simulink model "model_groundTethered"  (R2015b)
settings: Solver=ode45  StartTime=0.0  StopTime=T_sim  FixedStep=dt  RelTol=1e-3
PreLoadFcn:
  | setup;
InitFcn:
  | setup;
StartFcn:
  | setup;
values from neighbouring files (symbols this model uses):
  A_act = [-100 0 0 0 0 -100 0 0 0 0 -100 0 ... (16 elements, 4x4)]    [CD_spline.mat]    (also in CL_spline.mat; setup.m = -100*eye(4); setup_tmp_1p.m = -100*eye(4); setup_tmp_4p.m = -100*eye(4))
  A_init = [1.0386 0 12.9]    [CD_spline.mat]    (also in CL_spline.mat; setup_KiteModel_4points.m = Pc_init + d_n_r * w_k * w_rel * [-1;0;0])
  A_Kite = 7    [CD_spline.mat]    (also in CL_spline.mat; setup.m = 10.18; setup_tmp_1p.m = 10.18; setup_tmp_4p.m = 10.18)
  A_prd = [0 0 0 -640 0 0 0 0 0 0 -640 0 ... (36 elements, 6x6)]    [CD_spline.mat]    (also in CL_spline.mat; setup.m = 1000 * A_M_aug; setup_tmp_1p.m = 1000 * A_M_aug; setup_tmp_4p.m = 1000 * A_M_aug)
  A_ref = [0 0 0 -10000 0 0 0 0 0 0 -10000 0 ... (36 elements, 6x6)]    [CD_spline.mat]    (also in CL_spline.mat; setup.m = zeros(6); setup_tmp_1p.m = zeros(6); setup_tmp_4p.m = zeros(6))
  A_t_ref_cl = [0 0 0 -0.64 0 0 0 0 0 0 -0.64 0 ... (36 elements, 6x6)]    [CD_spline.mat]    (also in CL_spline.mat; setup.m = A_t_ref; setup_tmp_1p.m = A_t_ref; setup_tmp_4p.m = A_t_ref)
  alpha_0 = 10 * pi/180    (= 0.174532925199)    [setup_KiteModel_4points.m]
  alpha_s_0 = 10 * pi/180    (= 0.174532925199)    [setup_KiteModel_4points.m]
  ASideRel = 0    [CD_spline.mat]    (also in CL_spline.mat; setup.m; setup_tmp_1p.m; setup_tmp_4p.m = 0.306)
  B_act = [100 0 0 0 0 100 0 0 0 0 100 0 ... (16 elements, 4x4)]    [CD_spline.mat]    (also in CL_spline.mat; setup.m = 100*eye(4); setup_tmp_1p.m = 100*eye(4); setup_tmp_4p.m = 100*eye(4))
  B_init = [0 0 15.13]    [CD_spline.mat]    (also in CL_spline.mat; setup_KiteModel_4points.m = Pc_init + h_kite * [0;0;1;])
  B_ref = [0 0 0 10000 0 0 0 0 0 0 10000 0 ... (18 elements, 6x3)]    [CD_spline.mat]    (also in CL_spline.mat; setup.m = zeros(6,3); setup_tmp_1p.m = zeros(6,3); setup_tmp_4p.m = zeros(6,3))
  B_t_ref_cl = [0 0 0 0.64 0 0 0 0 0 0 0.64 0 ... (18 elements, 6x3)]    [CD_spline.mat]    (also in CL_spline.mat)
  Bpbl = [0 0 0 1 0 0 0 0 0 0 1 0 ... (18 elements, 6x3)]    [CD_spline.mat]    (also in CL_spline.mat; setup.m = [zeros(3); eye(3)]; setup_tmp_1p.m = [zeros(3); eye(3)]; setup_tmp_4p.m = [zeros(3); eye(3)])
  c0 = 614000    [CD_spline.mat]    (also in CL_spline.mat; setup.m; setup_tmp_1p.m; setup_tmp_4p.m)
  C_A = [0 0.3 -1e-06 1 -0.3 0 1e-06 1 0 -0.3 -1e-06 1 ... (16 elements, 4x4)]    [CD_spline.mat]    (also in CL_spline.mat; setup.m = [0, -R, 0, R; setup_tmp_1p.m = [0, -R, 0, R; setup_tmp_4p.m = [0, -R, 0, R)
  C_A_inv = [0 -1.66666666667 -1.23358113847e-17 1.66666666667 1.66666666667 2.46716227694e-17 -1.66666666667 0 -250000 250000 -250000 250000 ... (16 elements, 4x4)]    [CD_spline.mat]    (also in CL_spline.mat; setup.m = C_A \eye(4); setup_tmp_1p.m = C_A \eye(4); setup_tmp_4p.m = C_A \eye(4))
  C_D_Kite = 0.05    [CD_spline.mat]    (also in CL_spline.mat; setup.m = 0.005; setup_tmp_1p.m = 0.005)
  C_init = [0 2.5965 12.9]    [CD_spline.mat]    (also in CL_spline.mat; setup_KiteModel_4points.m = Pc_init + 0.5 * w_k * w_rel * [0;1;0])
  C_L_Kite = 0.1    [CD_spline.mat]    (also in CL_spline.mat; setup.m = 0.01; setup_tmp_1p.m = 0.01)
  CD_spline_coefs = CD_spline.coefs    [setup_KiteModel_4points.m]
  CD_tether = 0.96    [CD_spline.mat]    (also in CL_spline.mat; setup.m; setup_tmp_1p.m; setup_tmp_4p.m)
  CL_spline_coefs = CL_spline.coefs    [setup_KiteModel_4points.m]
  d0 = 473    [CD_spline.mat]    (also in CL_spline.mat; setup.m; setup_tmp_1p.m; setup_tmp_4p.m)
  D_init = [0 -2.5965 12.9]    [CD_spline.mat]    (also in CL_spline.mat; setup_KiteModel_4points.m = Pc_init - 0.5 * w_k * w_rel * [0;1;0])
  d_tether = 0.004    [CD_spline.mat]    (also in CL_spline.mat; setup.m; setup_tmp_1p.m; setup_tmp_4p.m)
  delta_dead = 0.5    [CD_spline.mat]    (also in CL_spline.mat; setup.m; setup_tmp_1p.m; setup_tmp_4p.m)
  e_0 = 0.01    [CD_spline.mat]    (also in CL_spline.mat; setup.m; setup_tmp_1p.m; setup_tmp_4p.m)
  epsilon = 0.6    [CD_spline.mat]    (also in CL_spline.mat; setup.m; setup_tmp_1p.m; setup_tmp_4p.m)
  eta_init = [0 0 0]    [CD_spline.mat]    (also in CL_spline.mat; setup.m = zeros(3,1); setup_tmp_1p.m = zeros(3,1); setup_tmp_4p.m = zeros(3,1))
  g = 9.81    [CD_spline.mat]    (also in CL_spline.mat; setup.m; setup_tmp_1p.m; setup_tmp_4p.m)
  g_vec = [0 0 9.81]    [CD_spline.mat]    (also in CL_spline.mat; setup.m = [0;0;9.81]; setup_tmp_1p.m = [0;0;9.81]; setup_tmp_4p.m = [0;0;9.81])
  Gamma_ad = 100    [CD_spline.mat]    (also in CL_spline.mat; setup.m = 100;100; setup_tmp_1p.m = 100;100; setup_tmp_4p.m = 100;100)
  Gamma_pred = 100    [CD_spline.mat]    (also in CL_spline.mat; setup.m; setup_tmp_1p.m; setup_tmp_4p.m)
  J = [0.018  0  0; 0  0.018  0; 0  0  0.009]    [CD_spline.mat]    (also in CL_spline.mat; setup.m = diag([Ixx, Iyy, Izz]); setup_tmp_1p.m = diag([Ixx, Iyy, Izz]); setup_tmp_4p.m = diag([Ixx, Iyy, Izz]))
  Jinv = [55.5555555556  0  0; 0  55.5555555556  0; 0  0  111.111111111]    [CD_spline.mat]    (also in CL_spline.mat; setup.m = J \ eye(3); setup_tmp_1p.m = J \ eye(3); setup_tmp_4p.m = J \ eye(3))
  K = 1 - ASideRel    [setup_KiteModel_4points.m]
  k_e_eta = 10000    [CD_spline.mat]    (also in CL_spline.mat; setup.m; setup_tmp_1p.m; setup_tmp_4p.m)
  k_e_eta_dot = 400    [CD_spline.mat]    (also in CL_spline.mat; setup.m; setup_tmp_1p.m; setup_tmp_4p.m)
  k_e_eta_I = 1    [CD_spline.mat]    (also in CL_spline.mat; setup.m; setup_tmp_1p.m; setup_tmp_4p.m)
  K_i_t = [10  0  0; 0  10  0; 0  0  10]    [CD_spline.mat]    (also in CL_spline.mat; setup.m = 10*eye(3); setup_tmp_1p.m = 10*eye(3); setup_tmp_4p.m = 10*eye(3))
  K_v_t = [1.6  0  0; 0  1.6  0; 0  0  1.6]    [CD_spline.mat]    (also in CL_spline.mat; setup.m = 2*omega_0_trans*zeta_0_trans*eye(3); setup_tmp_1p.m = 2*omega_0_trans*zeta_0_trans*eye(3); setup_tmp_4p.m = 2*omega_0_trans*zeta_0_trans*eye(3))
  K_x_t = [0.64  0  0; 0  0.64  0; 0  0  0.64]    [CD_spline.mat]    (also in CL_spline.mat; setup.m = omega_0_trans^2*eye(3); setup_tmp_1p.m = omega_0_trans^2*eye(3); setup_tmp_4p.m = omega_0_trans^2*eye(3))
  l_s0 = 1    [CD_spline.mat]    (also in CL_spline.mat; setup.m = 1.42857142857; setup_tmp_1p.m = 1.42857142857; setup_tmp_4p.m = 1.66666666667)
  l_s_BP = norm( B_init - p_B_UAV_init)    [setup_KiteModel_4points.m]
  l_s_PUav = norm( pos_UAV_init - p_B_UAV_init)    [setup_KiteModel_4points.m]
  ls_AB = norm( A_init -  B_init)    [setup_KiteModel_4points.m]
  ls_AC = norm( A_init -  C_init)    [setup_KiteModel_4points.m]
  ls_AD = norm( A_init -  D_init)    [setup_KiteModel_4points.m]
  ls_AKcu = norm( A_init -  P_kcu)    [setup_KiteModel_4points.m]
  ls_CB = norm( C_init -  B_init)    [setup_KiteModel_4points.m]
  ls_CD = norm( C_init -  D_init)    [setup_KiteModel_4points.m]
  ls_CKcu = norm( C_init - P_kcu)    [setup_KiteModel_4points.m]
  ls_DB = norm( D_init - B_init )    [setup_KiteModel_4points.m]
  ls_DKcu = norm( D_init - P_kcu)    [setup_KiteModel_4points.m]
  m_A = 3.29    [CD_spline.mat]    (also in CL_spline.mat; setup_KiteModel_4points.m = nose_mass_fraction * m_kite)
  m_B = 1.484    [CD_spline.mat]    (also in CL_spline.mat; setup_KiteModel_4points.m = 0.4 * (1-nose_mass_fraction)*m_kite)
  m_C = 1.113    [CD_spline.mat]    (also in CL_spline.mat; setup_KiteModel_4points.m = 0.3 * (1-nose_mass_fraction)*m_kite)
  m_D = 1.113    [CD_spline.mat]    (also in CL_spline.mat; setup_KiteModel_4points.m = 0.3 * (1-nose_mass_fraction)*m_kite)
  m_kite = 7    [CD_spline.mat]    (also in CL_spline.mat; setup.m = 5;7; setup_tmp_1p.m = 5;7; setup_tmp_4p.m = 6.21)
  m_p = 0.013    [CD_spline.mat]    (also in CL_spline.mat; setup.m = 0.0185714285714; setup_tmp_1p.m = 0.0185714285714; setup_tmp_4p.m = 0.0216666666667)
  m_uav = 3    [CD_spline.mat]    (also in CL_spline.mat; setup.m; setup_tmp_1p.m; setup_tmp_4p.m)
  n = 10    [CD_spline.mat]    (also in CL_spline.mat; setup.m; setup_tmp_1p.m; setup_tmp_4p.m)
  n_t_p = 7    [setup.m]    (also in setup_tmp_1p.m; setup_tmp_4p.m = 6)
  omega_init = [0 0 0]    [CD_spline.mat]    (also in CL_spline.mat; setup.m = zeros(3,1); setup_tmp_1p.m = zeros(3,1); setup_tmp_4p.m = zeros(3,1))
  p_B_UAV_init = B_init + [0;0;l_s0]    [setup_KiteModel_4points.m]
  p_init = [0 0 1 0 0 2 0 0 3 0 0 4 ... (30 elements, 30x1)]    [CD_spline.mat]    (also in CL_spline.mat; setup.m = zeros(3*n,1); setup_tmp_1p.m = zeros(3*n,1); setup_tmp_4p.m = zeros(3*n,1))
  p_init_4p = zeros(3*n_t_p,1)    [setup.m]    (also in setup_tmp_4p.m)
  P_prd = [712.5 0 0 156.25 0 0 0 712.5 0 0 156.25 0 ... (36 elements, 6x6)]    [CD_spline.mat]    (also in CL_spline.mat; setup.m = 1000 * P_tref; setup_tmp_1p.m = 1000 * P_tref; setup_tmp_4p.m = 1000 * P_tref)
  P_tref = [0.7125 0 0 0.15625 0 0 0 0.7125 0 0 0.15625 0 ... (36 elements, 6x6)]    [CD_spline.mat]    (also in CL_spline.mat; setup.m = lyap(A_M_aug', Q); setup_tmp_1p.m = lyap(A_M_aug', Q); setup_tmp_4p.m = lyap(A_M_aug', Q))
  pos_UAV_init = p_B_UAV_init + [0;0;l_s0]    [setup_KiteModel_4points.m]
  rho_air = 1.225    [CD_spline.mat]    (also in CL_spline.mat; setup.m; setup_tmp_1p.m; setup_tmp_4p.m)
  rho_t = 0.013    [CD_spline.mat]    (also in CL_spline.mat; setup.m; setup_tmp_1p.m; setup_tmp_4p.m)
  sample_log = 0.01    [CD_spline.mat]    (also in CL_spline.mat; setup.m; setup_tmp_1p.m; setup_tmp_4p.m)
  t0 = 1    [CD_spline.mat]    (also in CL_spline.mat; setup.m; setup_tmp_1p.m; setup_tmp_4p.m)
  t1 = 3    [CD_spline.mat]    (also in CL_spline.mat; setup.m; setup_tmp_1p.m; setup_tmp_4p.m)
  T_launch = 40    [CD_spline.mat]    (also in CL_spline.mat; setup.m; setup_tmp_1p.m; setup_tmp_4p.m)
  Theta_max = 60    [CD_spline.mat]    (also in CL_spline.mat; setup.m; setup_tmp_1p.m; setup_tmp_4p.m)
  Thrust_Max = 80    [CD_spline.mat]    (also in CL_spline.mat; setup.m = 1000000000; setup_tmp_1p.m = 100; setup_tmp_4p.m = 1000000000)
  Tx = 10    [CD_spline.mat]    (also in CL_spline.mat; setup.m; setup_tmp_1p.m; setup_tmp_4p.m)
  Ty = 10    [CD_spline.mat]    (also in CL_spline.mat; setup.m; setup_tmp_1p.m; setup_tmp_4p.m)
  Tz = 10    [CD_spline.mat]    (also in CL_spline.mat; setup.m; setup_tmp_1p.m; setup_tmp_4p.m = 15)
  v_w_vec = [1 1 1]    [CD_spline.mat]    (also in CL_spline.mat; setup.m = [0.1;0;0]; setup_tmp_1p.m = [1;0;0]; setup_tmp_4p.m = [3;0;0])
  x0num = 0    [CD_spline.mat]    (also in CL_spline.mat; polynomial_trajectory.m = double( solutions_x.x0 ))
  x1num = 0    [CD_spline.mat]    (also in CL_spline.mat; polynomial_trajectory.m = double( solutions_x.x1 ))
  x2num = 0    [CD_spline.mat]    (also in CL_spline.mat; polynomial_trajectory.m = double( solutions_x.x2 ))
  x3num = 0.05    [CD_spline.mat]    (also in CL_spline.mat; polynomial_trajectory.m = double( solutions_x.x3 ))
  x4num = -0.0075    [CD_spline.mat]    (also in CL_spline.mat; polynomial_trajectory.m = double( solutions_x.x4 ))
  x5num = 0.0003    [CD_spline.mat]    (also in CL_spline.mat; polynomial_trajectory.m = double( solutions_x.x5 ))
  x_drone_init = [0 0 10]    [CD_spline.mat]    (also in CL_spline.mat; setup.m = p_init(3*n-2:3*n); setup_KiteModel_4points.m = pos_UAV_init; setup_tmp_1p.m = p_init(3*n-2:3*n))
  xT = 5    [CD_spline.mat]    (also in CL_spline.mat; setup.m = 1; setup_tmp_1p.m = 10; setup_tmp_4p.m = 10)
  y0num = 0    [CD_spline.mat]    (also in CL_spline.mat; polynomial_trajectory.m = double( solutions_y.y0 ))
  y1num = 0    [CD_spline.mat]    (also in CL_spline.mat; polynomial_trajectory.m = double( solutions_y.y1 ))
  y2num = 0    [CD_spline.mat]    (also in CL_spline.mat; polynomial_trajectory.m = double( solutions_y.y2 ))
  y3num = 0.1    [CD_spline.mat]    (also in CL_spline.mat; polynomial_trajectory.m = double( solutions_y.y3 ))
  y4num = -0.015    [CD_spline.mat]    (also in CL_spline.mat; polynomial_trajectory.m = double( solutions_y.y4 ))
  y5num = 0.0006    [CD_spline.mat]    (also in CL_spline.mat; polynomial_trajectory.m = double( solutions_y.y5 ))
  yT = 10    [CD_spline.mat]    (also in CL_spline.mat; setup.m = 1; setup_tmp_1p.m = 0; setup_tmp_4p.m = 0)
  z0num = 10    [CD_spline.mat]    (also in CL_spline.mat; polynomial_trajectory.m = double( solutions_z.z0 ))
  z1num = 0    [CD_spline.mat]    (also in CL_spline.mat; polynomial_trajectory.m = double( solutions_z.z1 ))
  z2num = 0    [CD_spline.mat]    (also in CL_spline.mat; polynomial_trajectory.m = double( solutions_z.z2 ))
  z3num = 0.4    [CD_spline.mat]    (also in CL_spline.mat; polynomial_trajectory.m = double( solutions_z.z3 ))
  z4num = -0.06    [CD_spline.mat]    (also in CL_spline.mat; polynomial_trajectory.m = double( solutions_z.z4 ))
  z5num = 0.0024    [CD_spline.mat]    (also in CL_spline.mat; polynomial_trajectory.m = double( solutions_z.z5 ))
  zT = 50    [CD_spline.mat]    (also in CL_spline.mat; setup.m; setup_tmp_1p.m; setup_tmp_4p.m = 75)
libraries: simulink x1
(part 3 of 3)

== matlab function model_groundTethered/Controller/Outer_Loop_Position/Adaptive_Augmentation/Proj(Theta_hat, GammaY)_multicolumns/Projection_Input_1/calculate_gradf ==
  data: theta_hat input; gradf output; Theta_max input; epsilon input
function gradf = fcn(theta_hat,Theta_max, epsilon )
%#codegen
gradf = ( 2*(1+epsilon) ) / (epsilon*(Theta_max)^2) * theta_hat ;

== matlab function model_groundTethered/Controller/Pseudo_Control_Hedging/Rotate thrust vector according to attitude ==
  data: u_Thrust_I input; eta input; u_Thrust_B output
function u_Thrust_B   = thrust_Bz_direction(  u_Thrust_I, eta) 

phi = eta(1); 
theta = eta(2); 
psi = eta(3); 

% Rotate thrust vector such that it is perpendicular to the "rotor blades"
u_Thrust_B = [cos(psi)*cos(theta), sin(psi)*cos(theta), -sin(theta); 
            cos(psi)*sin(theta)*sin(phi)-sin(psi)*cos(phi), sin(psi)*sin(theta)*sin(phi)+cos(psi)*cos(phi), cos(theta)*sin(phi); 
            cos(psi)*sin(theta)*cos(phi)+sin(psi)*sin(phi), sin(psi)*sin(theta)*cos(phi)-cos(psi)*sin(phi), cos(theta)*cos(phi)] *...
            [0;0;u_Thrust_I];

== matlab function model_groundTethered/Controller/Pseudo_Control_Hedging/Plant_Inversion_RD2_backwards/Plant_Inversion ==
  data: omega input; nu_tot_rot_hat output; eta input; eta_dot input; J parameter; Jinv parameter; M_hat input
function nu_tot_rot_hat = fcn(omega, eta, eta_dot,J, Jinv, M_hat)
%#codegen
p = omega(1); 
q = omega(2); 
r = omega(3); 
Ix = J(1,1); 
Iy = J(2,2); 
Iz = J(3,3); 


cross_coupling = [ Iy*q*r - Iz*q*r
 Iz*p*r - Ix*p*r;
 Ix*p*q - Iy*p*q];

% T_inv = [1, sin(eta(1)) * tan(eta(2)), cos(eta(1)) * tan(eta(2)) ; 
% 0, cos(eta(1)), -sin(eta(1)); 
% 0, sin(eta(1))/cos(eta(2)), cos(eta(1))/cos(eta(2))] \ eye(3); 

T = [1, sin(eta(1)) * tan(eta(2)), cos(eta(1)) * tan(eta(2)) ; 
0, cos(eta(1)), -sin(eta(1)); 
0, sin(eta(1))/cos(eta(2)), cos(eta(1))/cos(eta(2))];

T_dot = eta_dot(1) * [0, cos(eta(1)) * tan(eta(2)), -sin(eta(1))*tan(eta(2)); 
                      0, -sin(eta(1)), -cos(eta(1));
                      0, cos(eta(1))/cos(eta(2)), -sin(eta(1))/cos(eta(2))]+...
        eta_dot(2) * [0, sin(eta(1))/cos(eta(2))^2, cos(eta(1))/cos(eta(2))^2; 
                       0, 0, 0; 
                       0, sin(eta(1))*sin(eta(2))/cos(eta(2))^2, cos(eta(1))*sin(eta(2))/cos(eta(2))^2];
                          
%u_NDI = -cross_coupling + J * T_inv * ( -T_dot * omega + nu_tot); 

nu_tot_rot_hat = T * Jinv * ( M_hat + cross_coupling ) + T_dot *omega;

== matlab function model_groundTethered/Controller/Pseudo_Control_Hedging/Plant_Inversion_RD2_backwards/estimate_eta_dot ==
  data: omega input; eta input; eta_dot output
function eta_dot  = fcn( omega, eta)
%#codegen

eta_dot = [1, sin(eta(1)) * tan(eta(2)), cos(eta(1)) * tan(eta(2)) ; 
0, cos(eta(1)), -sin(eta(1)); 
0, sin(eta(1))/cos(eta(2)), cos(eta(1))/cos(eta(2))] * omega;

== matlab function model_groundTethered/Controller/Outer_Loop_Position/Adaptive_Augmentation/Smooth_Deadzone_MRAC/smooth_deadzone ==
  data: e_norm input; mu_dead output; delta_dead input; e_0 input
function mu_dead = fcn(e_norm, delta_dead, e_0)
%#codegen

mu_dead = max( 0, min( 1, (e_norm - delta_dead*e_0)/...
                          ( (1-delta_dead) * e_0) ) );

== matlab function model_groundTethered/Controller/Outer_Loop_Position/Calc_Ref_Attitude ==
  data: T_ref input; Eta_Cmd output; eta input
function Eta_Cmd  = fcn(T_ref, eta)
%#codegen
psi = eta(3); 
theta = eta(2); 
phi = eta(1); 

psi_c = 0;

T = norm( T_ref ); 

phi_c = -asin( 1/T * (T_ref(1) * sin(psi_c) - T_ref(2) * cos(psi_c)) ); 
theta_c = -atan( 1/T_ref(3) * (T_ref(1) * cos(psi_c) + T_ref(2) * sin(psi_c))); 

Eta_Cmd = [phi_c;theta_c; 0];

== matlab function model_groundTethered/Plant/Tether_Kite_Tether_UAV_Dynamics_4P/Kite_Model_4p/Kite_Model_4p ==
  data: x_dotdot_kite output; v_w_vec input; ASideRel parameter; alpha_d input; alpha_0 parameter; alpha_s input; alpha_s_0 parameter; x_kite_A input; x_kite_B input; x_kite_C input; x_kite_D input; x_kite_kcu input; x_above_kite input; xdot_kite_A input; xdot_kite_B input; xdot_kite_C input; xdot_kite_D input; xdot_kite_kcu input; xdot_above_kite input; CL_spline_coefs parameter; CD_spline_coefs parameter; rho_air parameter; A_Kite parameter; K parameter; g_vec parameter; m_A parameter; m_B parameter; m_C parameter; m_D parameter; d0 parameter; c0 parameter; ls_AC parameter; ls_AB parameter; ls_AKcu parameter; ls_AD parameter; ls_CB parameter; ls_CD parameter; ls_CKcu parameter; ls_DKcu parameter; ls_DB parameter; l_s_BP parameter
%% 4 Point kite implementation

function x_dotdot_kite  = fcn( v_w_vec, ASideRel, alpha_d,alpha_0,alpha_s, alpha_s_0,...
    x_kite_A, x_kite_B, x_kite_C, x_kite_D, x_kite_kcu,...
    x_above_kite, xdot_kite_A, xdot_kite_B, xdot_kite_C, xdot_kite_D,xdot_kite_kcu,xdot_above_kite,...
    CL_spline_coefs, CD_spline_coefs, rho_air, A_Kite,K,g_vec, m_A, m_B, m_C, m_D, d0, c0,...
    ls_AC, ls_AB, ls_AKcu, ls_AD, ls_CB, ls_CD, ls_CKcu, ls_DKcu, ls_DB,l_s_BP )


% Calculation of unity vectors of the kite body fixed frame
x_kite_Pc = 0.5 * (x_kite_C + x_kite_D);
e_z_k = (x_kite_Pc - x_kite_B)/sqrt((x_kite_Pc - x_kite_B)'*(x_kite_Pc - x_kite_B));
e_y_k = (x_kite_C - x_kite_D)/sqrt((x_kite_C - x_kite_D)'*(x_kite_C - x_kite_D));
e_x_k = [ e_y_k(2)*e_z_k(3) - e_y_k(3)*e_z_k(2);
    e_y_k(3)*e_z_k(1) - e_y_k(1)*e_z_k(3);
    e_y_k(1)*e_z_k(2) - e_y_k(2)*e_z_k(1)];

% Calculation of the apparent wind speeds at the 3 lifting surfaces
v_a_k_B = v_w_vec - xdot_kite_B;
v_a_k_C = v_w_vec - xdot_kite_C;
v_a_k_D = v_w_vec - xdot_kite_D;

% Calculation of the apparent wind speeds in xy and xz plane
v_a_B_xz = v_a_k_B - (v_a_k_B'*e_y_k)*e_y_k;
v_a_C_xy = v_a_k_C - (v_a_k_C'*e_z_k)*e_z_k;
v_a_D_xy = v_a_k_D - (v_a_k_D'*e_z_k)*e_z_k;

% Calculation of angles of attack
alpha_B  = pi - acos( (v_a_B_xz'*e_x_k)/sqrt(v_a_B_xz'*v_a_B_xz) ) - alpha_d + alpha_0;
alpha_C  = pi - acos( (v_a_C_xy'*e_x_k)/sqrt(v_a_C_xy'*v_a_C_xy) ) - alpha_s + alpha_s_0;
alpha_D  = pi - acos( (v_a_D_xy'*e_x_k)/sqrt(v_a_D_xy'*v_a_D_xy) ) + alpha_s + alpha_s_0;

% Calculation of Cl(alpha)_i and Cd(alpha)_i based on the spline
% coefficients
[ C_L_B, C_D_B ] = calcCLandCD_4pKite( alpha_B,CL_spline_coefs,CD_spline_coefs );
[ C_L_C, C_D_C ] = calcCLandCD_4pKite( alpha_C,CL_spline_coefs,CD_spline_coefs );
[ C_L_D, C_D_D ] = calcCLandCD_4pKite( alpha_D,CL_spline_coefs,CD_spline_coefs);

% Calculate the lift and drag forces of the lifting surfaces
[ F_L_B, F_L_C, F_L_D,...
    F_D_B, F_D_C, F_D_D  ] = calc4pKiteForces( C_L_B,C_L_C,C_L_D,...
    C_D_B, C_D_C, C_D_D,...
    rho_air, A_Kite, ASideRel,K,...
    e_y_k, e_z_k,...
    v_a_k_B, v_a_k_C, v_a_k_D, ...
    v_a_B_xz, v_a_C_xy, v_a_D_xy);

% Spring-Damper forces 
% Constant bridle line (as defined in the setup_KiteModel_4points.m script)
% Notation: z.B. AC => x_A - x_C => belongs to forces of inertia

c = c0;
d = d0;

f_AC = calcSpringDamperForce(c, norm(x_kite_A-x_kite_C) , ls_AC, d, x_kite_A - x_kite_C, xdot_kite_A - xdot_kite_C, 1 );
f_AB = calcSpringDamperForce(c, norm(x_kite_A-x_kite_B) , ls_AB, d, x_kite_A - x_kite_B, xdot_kite_A - xdot_kite_B, 1 );
f_AD = calcSpringDamperForce(c, norm(x_kite_A-x_kite_D) , ls_AD, d, x_kite_A - x_kite_D, xdot_kite_A - xdot_kite_D, 1 );
f_A_kcu = calcSpringDamperForce(c, norm(x_kite_A-x_kite_kcu) , ls_AKcu, d, x_kite_A - x_kite_kcu, xdot_kite_A - xdot_kite_kcu, 1 );
f_CA = -f_AC; 
f_CD = calcSpringDamperForce(c, norm(x_kite_C-x_kite_D) , ls_CD, d, x_kite_C - x_kite_D, xdot_kite_C - xdot_kite_D, 1 ); 
f_CB = calcSpringDamperForce(c, norm(x_kite_C-x_kite_B) , ls_CB, d, x_kite_C - x_kite_B, xdot_kite_C - xdot_kite_B, 1 ); 
f_C_kcu = calcSpringDamperForce(c, norm(x_kite_C-x_kite_kcu) , ls_CKcu, d, x_kite_C - x_kite_kcu, xdot_kite_C - xdot_kite_kcu, 1 );
f_DA = -f_AD; 
f_DC = -f_CD; 
f_DB = calcSpringDamperForce(c, norm(x_kite_D-x_kite_B) , ls_DB, d, x_kite_D - x_kite_B, xdot_kite_D - xdot_kite_B, 1 ); 
f_D_kcu = calcSpringDamperForce(c, norm(x_kite_D-x_kite_kcu) , ls_DKcu, d, x_kite_D - x_kite_kcu, xdot_kite_D - xdot_kite_kcu, 1 );
f_BA = -f_AB; 
f_BC = -f_CB; 
f_BD = -f_DB;  
f_above_kite = calcSpringDamperForce(c0, norm(x_above_kite-x_kite_B) , l_s_BP, d0, x_above_kite - x_kite_B, xdot_above_kite - xdot_kite_B, 1 ); 

x_kite_A_dotdot = 1/m_A*( - m_A*g_vec - f_AC - f_AB - f_A_kcu );
x_kite_B_dotdot = 1/m_B*(F_L_B + F_D_B - m_B*g_vec - f_BA - f_BC - f_BD + f_above_kite  );
x_kite_C_dotdot = 1/m_C*(F_L_C + F_D_C - m_C*g_vec - f_CA - f_CD - f_CB - f_C_kcu );
x_kite_D_dotdot = 1/m_D*(F_L_D + F_D_D - m_D*g_vec - f_DA - f_DC - f_DB - f_D_kcu );

x_dotdot_kite = [x_kite_A_dotdot;
                 x_kite_B_dotdot;
                 x_kite_C_dotdot;
                 x_kite_D_dotdot];

end

== matlab function model_groundTethered/Plant/Tether_Kite_Tether_UAV_Dynamics_1P/Kite_Model_1P/Kite_Model ==
  data: launch_flag input; x_dotdot_kite output; rho_air parameter; A_Kite parameter; g_vec parameter; C_L_Kite parameter; C_D_Kite parameter; m_kite parameter; v_w_vec input; ASideRel parameter; xp_aboveKite input; x_kite input; xp_belowKite input; xdot_aboveKite input; xdot_kite input; xdot_belowKite input; l_s input; c0 parameter; d0 parameter; l_s0 parameter
function x_dotdot_kite  = fcn(launch_flag,...
    rho_air, A_Kite, g_vec, C_L_Kite, C_D_Kite, m_kite, v_w_vec, ASideRel,...
    xp_aboveKite, x_kite, xp_belowKite,xdot_aboveKite, xdot_kite,...
    xdot_belowKite, l_s, c0, d0, l_s0)

c = c0/l_s;
d = d0/l_s;

% Tether forces from below and above
f_T_below = calcSpringDamperForce(c, norm(x_kite-xp_belowKite) , l_s, d, x_kite - xp_belowKite, xdot_kite - xdot_belowKite, 1 );
f_T_above = calcSpringDamperForce(c0, norm(xp_aboveKite-x_kite), l_s0, d0, xp_aboveKite-x_kite, xdot_aboveKite - xdot_kite, 1 );

% Calculate the apparent wind speed
v_a_k = v_w_vec - xdot_kite;
if launch_flag
    C_L_Kite = 0.5;
    C_D_Kite = 0.2;
end

[L_kite, D_kite, S_kite] = calcKiteForces(x_kite, xp_belowKite, ...
                                        v_a_k, C_L_Kite, rho_air, A_Kite, C_D_Kite, ASideRel);
m_kite = 0.1;
if launch_flag % kite is launched
    x_dotdot_kite = 1/m_kite * ( -f_T_below  - m_kite*g_vec  ... % remove the conection to 'drone tether'
        + D_kite + L_kite + 0*S_kite ) ;  % Kite dynamics
else
    x_dotdot_kite = 1/m_kite * ( -f_T_below + f_T_above - m_kite*g_vec  ...
        + 0*D_kite + 0*L_kite  + 0*S_kite);  % Kite dynamics
end

== matlab function model_groundTethered/Plant/Tether_Kite_Tether_UAV_Dynamics_4P/UAV_Model/Rotate thrust vector according to attitude ==
  data: u_Thrust_I input; eta input; u_Thrust_B output
function u_Thrust_B   = thrust_Bz_direction(  u_Thrust_I, eta) 

phi = eta(1); 
theta = eta(2); 
psi = eta(3); 

% Rotate thrust vector such that it is perpendicular to the "rotor blades"
u_Thrust_B = [cos(psi)*cos(theta), sin(psi)*cos(theta), -sin(theta); 
            cos(psi)*sin(theta)*sin(phi)-sin(psi)*cos(phi), sin(psi)*sin(theta)*sin(phi)+cos(psi)*cos(phi), cos(theta)*sin(phi); 
            cos(psi)*sin(theta)*cos(phi)+sin(psi)*sin(phi), sin(psi)*sin(theta)*cos(phi)-cos(psi)*sin(phi), cos(theta)*cos(phi)] *...
            [0;0;u_Thrust_I];

== matlab function model_groundTethered/Controller/Outer_Loop_Position/Adaptive_Augmentation/Proj(Theta_hat, GammaY)_1column/Proj(Theta,Theta_dot) ==
  data: flag output; f input; gradf input; Theta_dot input; Theta_hat_dot_ output; direction output; orthogonal_part output
function  [flag,Theta_hat_dot_, direction, orthogonal_part] = fcn(f, gradf, Theta_dot )
%#codegen


if ( f > 0 && Theta_dot'*gradf > 0 )
    flag  = 1;
    direction = Theta_dot'*gradf;
    Theta_hat_dot_ = Theta_dot - f * ( (gradf*gradf') / (gradf'*gradf) * Theta_dot )   ;
    orthogonal_part = f * ( (gradf*gradf') / (gradf'*gradf) * Theta_dot );
else
    direction = Theta_dot'*gradf;
    flag = 0;
    Theta_hat_dot_ =  Theta_dot;
    orthogonal_part = zeros(3,1);
end

== matlab function model_groundTethered/Controller/Outer_Loop_Position/Adaptive_Augmentation/Proj(Theta_hat, GammaY)_1column/calculate_f ==
  data: theta_hat input; f output; Theta_max input; epsilon input
function f   = fcn(theta_hat,Theta_max, epsilon )
%#codegen
f = ( (1+epsilon)*norm(theta_hat)^2 - (Theta_max)^2 ) / (epsilon*(Theta_max)^2);

== matlab function model_groundTethered/Controller/Outer_Loop_Position/Adaptive_Augmentation/Proj(Theta_hat, GammaY)_1column/calculate_gradf ==
  data: theta_hat input; gradf output; Theta_max input; epsilon input
function gradf = fcn(theta_hat,Theta_max, epsilon )
%#codegen
gradf = ( 2*(1+epsilon) ) / (epsilon*(Theta_max)^2) * theta_hat ;

== matlab function model_groundTethered/Controller/Reelout_Speed_Control/Activation_Function ==
  data: d input; safety_factor_vro output
function safety_factor_vro = fcn(d)
%#codegen
zero_cross = 0.5;
% Sigmoid like function. Converges against 1 if d > zero_cross
% and against -1 if d < zero_cross. It is used to ensure that the 
% current tether length cannot enter the "safety-ball" around the drone.
safety_factor_vro = 2*( 1 ./ ( 1 + exp(-5*( d - zero_cross ) ) ) - 0.5 ) ;

== matlab function model_groundTethered/Analysis/Evaluate_Lyapunovfunction ==
  data: xi input; V output; P input; d_hat input; gamma_d input; e_pred input; P_pred input; d_real input
function V = fcn(xi, P, d_hat, gamma_d, e_pred, P_pred,d_real)
%#codegen
d_real = [5;5;5];
d_tilde = -d_hat - d_real;
V = 0.5 * xi' * P * xi + ...
    0.5 * e_pred * P_pred * e_pred' + ...
    0.5 * trace(d_tilde * 1 / gamma_d * d_tilde');

== matlab function model_groundTethered/Plant/Tether_Kite_Tether_UAV_Dynamics_4P/Tethermodel_Kite2UAV/Tether_Kite2UAV ==
  data: launch_flag input; x_dotdot_p output; m_p parameter; g_vec parameter; xp_above input; xp input; xp_below input; xp_dot_above input; xp_dot input; xp_dot_below input; c0 parameter; d0 parameter; l_s_PUav parameter; l_s_BP parameter; CD_tether parameter; d_tether parameter; rho_air parameter; v_w_vec input; f_T_below output; f_T_above output
function [x_dotdot_p,f_T_below,f_T_above]  = fcn(launch_flag, m_p, g_vec, xp_above, xp, xp_below, xp_dot_above, xp_dot, xp_dot_below,...
                        c0, d0, l_s_PUav, l_s_BP, CD_tether, d_tether, rho_air, v_w_vec  )
%#codegen
% Tether forces from below and above
f_T_below = calcSpringDamperForce(c0, norm(xp - xp_below) , l_s_BP, d0, xp - xp_below, xp_dot - xp_dot_below, 1 );
f_T_above = calcSpringDamperForce(c0, norm(xp_above - xp), l_s_PUav, d0, xp_above - xp, xp_dot_above - xp_dot, 1 );

v_a_p = v_w_vec - 0.5 * ( xp_dot + xp_dot_above ) ; 
Dp = calcSegmentDrag( xp_above - xp  , v_a_p, rho_air, CD_tether, d_tether );

if launch_flag
    x_dotdot_p = 1/m_p * ( f_T_above - m_p*g_vec  + Dp ); % Particle dynamics
else
    x_dotdot_p = 1/m_p * ( -f_T_below + f_T_above - m_p*g_vec  + Dp );  %
end

== matlab function model_groundTethered/Plant/Tether_Kite_Tether_UAV_Dynamics_4P/Tethermodel_Ground2Kite_4P/Tether_Ground2Kite ==
  data: x_dot input; x input; x_dotdot_TetherG2K output; v_w_vec input; d_tether parameter; CD_tether parameter; v_ro_set input; l_s input; c0 parameter; d0 parameter; rho_t parameter; g_vec parameter; rho_air parameter; l_tether output; l_s_dot output; x_kite_A input; x_kite_C input; x_kite_D input; xdot_kite_A input; xdot_kite_C input; xdot_kite_D input; ls_AKcu parameter; ls_CKcu parameter; ls_DKcu parameter
function [x_dotdot_TetherG2K,...
    l_tether, l_s_dot]    = fcn(x_dot, x,  v_w_vec,...
    d_tether, CD_tether, v_ro_set,l_s, c0, d0, rho_t, g_vec, rho_air,...
    x_kite_A,x_kite_C,x_kite_D ,xdot_kite_A,xdot_kite_C,xdot_kite_D, ls_AKcu, ls_CKcu,  ls_DKcu   )

%#codegen
n = 10;
n_t_p = 7; % amount of groudn particles
l_tether = l_s * n_t_p; % Tether length from ground to kite
l_s_dot = v_ro_set/n_t_p;

% Adapt stiffness and damping with respect to current segment length
c = c0/l_s;
d = d0/l_s;

% Mass of tether segments with  respect to current segment length
m = l_s * rho_t;
m_vec = m * ones(n_t_p,1);

p_vec = x;
v_vec = x_dot;
p_norm = zeros(n_t_p,1);

% Vector with distances between particles
p_d = p_vec - [0;0;0; p_vec(1:3*n_t_p-3)];

% Vector with velocity differences
v_d = v_vec - [0;0;0; v_vec(1:3*n_t_p-3)];

% calculate absolute distances between points
for iter = 1 : n_t_p
    p_norm(iter) = norm( p_d( (iter-1)* 3 + 1 : (iter-1) * 3 + 3 ) );
end

%%------------------------------- Equations of motions-------------------------------
% Initialize matrices
fsd_tot_mat = zeros(3,n_t_p);
x_dotdot = zeros(3,n_t_p);
D_s_mat = zeros(3,n_t_p);

%% Set up equations of motions of ground to kite tether

% Boundary tether force from kite to particle below kite (in the 4p kite model the kcu is connected to the
% points A, C and D

f_kite_A = calcSpringDamperForce( c0/ls_AKcu,norm( x_kite_A - p_vec(3*(n_t_p) -2 : 3*(n_t_p) ) ), ls_AKcu, d0/ls_AKcu,...
            x_kite_A - p_vec(3*(n_t_p) -2 : 3*(n_t_p) ) ,...
            xdot_kite_A - v_vec(3*(n_t_p)), 1 );
f_kite_C= calcSpringDamperForce( c0/ls_CKcu,norm( x_kite_C - p_vec(3*(n_t_p) -2 : 3*(n_t_p) ) ), ls_CKcu, d0/ls_CKcu,...
            x_kite_C - p_vec(3*(n_t_p) -2 : 3*(n_t_p) ) ,...
            xdot_kite_C - v_vec(3*(n_t_p)), 1 );
f_kite_D = calcSpringDamperForce( c0/ls_DKcu,norm( x_kite_D - p_vec(3*(n_t_p) -2 : 3*(n_t_p) ) ), ls_DKcu, d0/ls_DKcu,...
            x_kite_D - p_vec(3*(n_t_p) -2 : 3*(n_t_p) ) ,...
            xdot_kite_D - v_vec(3*(n_t_p)), 1 );        
        
        
for idx = 1 : n_t_p
    
    % Calculate Spring-Damper forces
    fsd_tot_mat(:,idx) = calcSpringDamperForce( c, p_norm(idx), l_s, d, p_d( (idx-1)*3+1:(idx-1)*3+3 ), v_d( (idx-1)*3+1:(idx-1)*3+3), idx );
    if idx < n_t_p
        fsd_tot_mat(:,idx+1) = calcSpringDamperForce( c, p_norm(idx+1), l_s, d, p_d( idx*3+1:idx*3+3 ), v_d( idx*3+1:idx*3+3), idx );       
    end
    
    % Calculate apparent wind speed of tether particles
    if idx == 1 % Segment that is connected to the ground
        v_a_p = v_w_vec - 0.5*x_dot(1:3) ;
    else
        v_a_p = v_w_vec - 0.5*( x_dot((idx-1)*3+1:(idx-1)*3+3) + x_dot((idx-1)*3:(idx-1)*3+2) ); % take mean value of adjacent particle vel. for segment velocity
    end
    
    % Calculate segment drag
    D_s_mat(:,idx) = calcSegmentDrag(p_d((idx-1)*3+1:(idx-1)*3+3) , v_a_p, rho_air, CD_tether, d_tether); % segment drag
    
    if idx < n_t_p
        % Equations of motion for the groud tether particles Newton x_dotdot = 1/m * (-f + u -mg )
        x_dotdot(:,idx) = 1/m_vec(idx) * ( -fsd_tot_mat(:,idx) + fsd_tot_mat(:,idx+1) - m_vec(idx)*g_vec  + D_s_mat(:,idx) );  % Particle dynamics
    else
        x_dotdot(:,idx) = 1/m_vec(idx) * ( -fsd_tot_mat(:,idx) + ...
            f_kite_A + f_kite_C + f_kite_D - m_vec(idx)*g_vec  + D_s_mat(:,idx) );  % Particle dynamics
    end
    
end


%% Reshape the structure of x_dotdot such that x_dotdot = [x1;y1;z1;x2;y2;...]
x_dotdot_TetherG2K = reshape(x_dotdot, [3*n_t_p,1]);

== matlab function model_groundTethered/Controller/Outer_Loop_Position/Adaptive_Augmentation/Proj(Theta_hat, GammaY)_multicolumns/Projection_Input_2/Proj(Theta,Theta_dot) ==
  data: f input; gradf input; Theta_dot input; Theta_hat_dot_ output
function  Theta_hat_dot_ = fcn(f, gradf, Theta_dot )
%#codegen


if ( f > 0 && gradf*Theta_dot' > 0 )
    Theta_hat_dot_ = Theta_dot - f * ( (gradf'*gradf) / (gradf*gradf') * Theta_dot' )'   ;
else
    Theta_hat_dot_ =  Theta_dot;
end

== matlab function model_groundTethered/Plant/Tether_Kite_Tether_UAV_Dynamics_4P/UAV_Model/UAV_Dynamics ==
  data: x_dotdot_uav_trans output; omega_dot output; eta_dot output; Thrust input; m_uav parameter; g_vec parameter; x_UAV input; x_below_UAV input; x_dot_UAV input; x_dot_belowUAV input; c0 parameter; d0 parameter; l_s0 parameter; disturbance output; omega input; u_M input; J parameter; Jinv parameter; eta input
function [x_dotdot_uav_trans,omega_dot, eta_dot,  disturbance] = fcn(Thrust, m_uav, g_vec, x_UAV, x_below_UAV, x_dot_UAV, x_dot_belowUAV,...
    c0, d0, l_s0, omega, u_M, J,Jinv,eta )
%#codegen

%% Translational Dynamics
f_T_below = calcSpringDamperForce(c0, norm(x_UAV-x_below_UAV) , l_s0, d0, x_UAV-x_below_UAV, x_dot_UAV - x_dot_belowUAV, 1 );
disturbance = -f_T_below/m_uav;
%disturbance = 1/m_uav *[0;0;25] ;
x_dotdot_uav_trans = 1/m_uav * ( -0*f_T_below + Thrust - m_uav*g_vec + 0*[0;0;25]  ) ; % Drone dynamics

%% Rotational Dynamics 
p = omega(1); 
q = omega(2); 
r = omega(3); 
Ix = J(1,1); 
Iy = J(2,2); 
Iz = J(3,3); 

cross_coupling = [ Iy*q*r - Iz*q*r
                   Iz*p*r - Ix*p*r;
                   Ix*p*q - Iy*p*q];
% Bodyrate Dynamics
omega_dot = Jinv * ( cross_coupling + u_M ) ;  

% Attitude Dynamics
eta_dot = [1, sin(eta(1)) * tan(eta(2)), cos(eta(1)) * tan(eta(2)) ; 
0, cos(eta(1)), -sin(eta(1)); 
0, sin(eta(1))/cos(eta(2)), cos(eta(1))/cos(eta(2))] * omega ;

== matlab function model_groundTethered/Controller/Outer_Loop_Position/Adaptive_Augmentation/Proj(Theta_hat, GammaY)_multicolumns/Projection_Input_2/calculate_f ==
  data: theta_hat input; f output; Theta_max input; epsilon input
function f   = fcn(theta_hat,Theta_max, epsilon )
%#codegen
f = ( (1+epsilon)*norm(theta_hat)^2 - (Theta_max)^2 ) / (epsilon*(Theta_max)^2);

== matlab function model_groundTethered/Controller/Outer_Loop_Position/Adaptive_Augmentation/Proj(Theta_hat, GammaY)_multicolumns/Projection_Input_2/calculate_gradf ==
  data: theta_hat input; gradf output; Theta_max input; epsilon input
function gradf = fcn(theta_hat,Theta_max, epsilon )
%#codegen
gradf = ( 2*(1+epsilon) ) / (epsilon*(Theta_max)^2) * theta_hat ;

== matlab function model_groundTethered/Controller/Outer_Loop_Position/Adaptive_Augmentation/Proj(Theta_hat, GammaY)_multicolumns/Projection_Input_3/Proj(Theta,Theta_dot) ==
  data: flag output; f input; gradf input; Theta_dot input; Theta_hat_dot_ output; direction output
function  [flag,Theta_hat_dot_, direction] = fcn(f, gradf, Theta_dot )
%#codegen


if ( f > 0 && gradf*Theta_dot' > 0 )
    flag  = 1;
    direction = gradf*Theta_dot';
    Theta_hat_dot_ = Theta_dot - f * ( (gradf'*gradf) / (gradf*gradf') * Theta_dot' )'   ;
else
    direction = gradf*Theta_dot';
    flag = 0;
    Theta_hat_dot_ =  Theta_dot;
end

== matlab function model_groundTethered/Controller/Outer_Loop_Position/Adaptive_Augmentation/Proj(Theta_hat, GammaY)_multicolumns/Projection_Input_3/calculate_f ==
  data: theta_hat input; f output; Theta_max input; epsilon input
function f   = fcn(theta_hat,Theta_max, epsilon )
%#codegen
f = ( (1+epsilon)*norm(theta_hat)^2 - (Theta_max)^2 ) / (epsilon*(Theta_max)^2);

== matlab function model_groundTethered/Controller/Outer_Loop_Position/Adaptive_Augmentation/Proj(Theta_hat, GammaY)_multicolumns/Projection_Input_3/calculate_gradf ==
  data: theta_hat input; gradf output; Theta_max input; epsilon input
function gradf = fcn(theta_hat,Theta_max, epsilon )
%#codegen
gradf = ( 2*(1+epsilon) ) / (epsilon*(Theta_max)^2) * theta_hat ;

== matlab function model_groundTethered/Plant/Tether_Kite_Tether_UAV_Dynamics_1P/Tethermodel_Ground2Kite_1P/Tether_Ground2Kite ==
  data: x_dot input; x input; x_dotdot_TetherG2K output; v_w_vec input; d_tether parameter; CD_tether parameter; v_ro_set input; l_s input; c0 parameter; d0 parameter; rho_t parameter; g_vec parameter; rho_air parameter; l_tether output; l_s_dot output; xp_kite input; xp_dot_kite input
function [x_dotdot_TetherG2K,...
    l_tether, l_s_dot]    = fcn(x_dot, x,  v_w_vec,...
    d_tether, CD_tether, v_ro_set,l_s, c0, d0, rho_t, g_vec, rho_air, xp_kite, xp_dot_kite )

%#codegen
n = 10;
n_t_p = n-3;
l_tether = l_s * (n_t_p+1); % Tether length from ground to kite
l_s_dot = v_ro_set/(n_t_p+1);

% Adapt stiffness and damping with respect to current segment length
c = c0/l_s;
d = d0/l_s;

% Mass of tether segments with  respect to current segment length
m = l_s * rho_t;
m_vec = m * ones(n_t_p,1);

p_vec = x;
v_vec = x_dot;
p_norm = zeros(n_t_p,1);

% Vector with distances between particles
p_d = p_vec - [0;0;0; p_vec(1:3*n_t_p-3)];

% Vector with velocity differences
v_d = v_vec - [0;0;0; v_vec(1:3*n_t_p-3)];

% calculate absolute distances between points
for iter = 1 : n_t_p
    p_norm(iter) = norm( p_d( (iter-1)* 3 + 1 : (iter-1) * 3 + 3 ) );
end

%%------------------------------- Equations of motions-------------------------------
% Initialize matrices
fsd_tot_mat = zeros(3,n_t_p);
x_dotdot = zeros(3,n_t_p);
D_s_mat = zeros(3,n_t_p);

%% Set up equations of motions of ground to kite tether

% Boundary tether force from kite to particle below kite
f_kite = calcSpringDamperForce( c,norm( xp_kite - p_vec(3*(n-3) -2 : 3*(n-3) ) ), l_s, d,...
            xp_kite - p_vec(3*(n-3) -2 : 3*(n-3) ) ,...
            xp_dot_kite - v_vec(3*(n-3)), 1 );
        
for idx = 1 : n_t_p
    
    % Calculate Spring-Damper forces
    fsd_tot_mat(:,idx) = calcSpringDamperForce( c, p_norm(idx), l_s, d, p_d( (idx-1)*3+1:(idx-1)*3+3 ), v_d( (idx-1)*3+1:(idx-1)*3+3), idx );
    if idx < n_t_p
        fsd_tot_mat(:,idx+1) = calcSpringDamperForce( c, p_norm(idx+1), l_s, d, p_d( idx*3+1:idx*3+3 ), v_d( idx*3+1:idx*3+3), idx );       
    end
    
    % Calculate apparent wind speed of tether particles
    if idx == 1 % Segment that is connected to the ground
        v_a_p = v_w_vec - 0.5*x_dot(1:3) ;
    else
        v_a_p = v_w_vec - 0.5*( x_dot((idx-1)*3+1:(idx-1)*3+3) + x_dot((idx-1)*3:(idx-1)*3+2) ); % take mean value of adjacent particle vel. for segment velocity
    end
    
    % Calculate segment drag
    D_s_mat(:,idx) = calcSegmentDrag(p_d((idx-1)*3+1:(idx-1)*3+3) , v_a_p, rho_air, CD_tether, d_tether); % segment drag
    
    if idx < n_t_p
        % Equations of motion for the groud tether particles Newton x_dotdot = 1/m * (-f + u -mg )
        x_dotdot(:,idx) = 1/m_vec(idx) * ( -fsd_tot_mat(:,idx) + fsd_tot_mat(:,idx+1) - m_vec(idx)*g_vec  + D_s_mat(:,idx) );  % Particle dynamics
    else
        x_dotdot(:,idx) = 1/m_vec(idx) * ( -fsd_tot_mat(:,idx) + f_kite - m_vec(idx)*g_vec  + D_s_mat(:,idx) );  % Particle dynamics
    end
    
end


%% Reshape the structure of x_dotdot such that x_dotdot = [x1;y1;z1;x2;y2;...]
x_dotdot_TetherG2K = reshape(x_dotdot, [3*n_t_p,1]);

== matlab function model_groundTethered/Plant/Tether_Kite_Tether_UAV_Dynamics_1P/Tethermodel_Kite2UAV/Tether_Kite2UAV ==
  data: launch_flag input; x_dotdot_p output; m_p parameter; g_vec parameter; xp_above input; xp input; xp_below input; xp_dot_above input; xp_dot input; xp_dot_below input; c0 parameter; d0 parameter; l_s0 parameter; CD_tether parameter; d_tether parameter; rho_air parameter; v_w_vec input
function x_dotdot_p = fcn(launch_flag, m_p, g_vec, xp_above, xp, xp_below, xp_dot_above, xp_dot, xp_dot_below,...
                        c0, d0, l_s0, CD_tether, d_tether, rho_air, v_w_vec  )
%#codegen
% Tether forces from below and above
f_T_below = calcSpringDamperForce(c0, norm(xp - xp_below) , l_s0, d0, xp - xp_below, xp_dot - xp_dot_below, 1 );
f_T_above = calcSpringDamperForce(c0, norm(xp_above - xp), l_s0, d0, xp_above - xp, xp_dot_above - xp_dot, 1 );

v_a_p = v_w_vec - 0.5 * ( xp_dot + xp_above ) ; % FALSE: has to be xp_dot + xp_dot_above !!!!
Dp = calcSegmentDrag( xp_above - xp  , v_a_p, rho_air, CD_tether, d_tether );

if launch_flag
    x_dotdot_p = 1/m_p * ( f_T_above - m_p*g_vec  + Dp ); % Particle dynamics
else
    x_dotdot_p = 1/m_p * ( -f_T_below + f_T_above - m_p*g_vec  + Dp );  %
end

== matlab function model_groundTethered/Plant/Tether_Kite_Tether_UAV_Dynamics_1P/UAV_Model/Rotate thrust vector according to attitude ==
  data: u_Thrust_I input; eta input; u_Thrust_B output
function u_Thrust_B   = thrust_Bz_direction(  u_Thrust_I, eta) 

phi = eta(1); 
theta = eta(2); 
psi = eta(3); 

% Rotate thrust vector such that it is perpendicular to the "rotor blades"
u_Thrust_B = [cos(psi)*cos(theta), sin(psi)*cos(theta), -sin(theta); 
            cos(psi)*sin(theta)*sin(phi)-sin(psi)*cos(phi), sin(psi)*sin(theta)*sin(phi)+cos(psi)*cos(phi), cos(theta)*sin(phi); 
            cos(psi)*sin(theta)*cos(phi)+sin(psi)*sin(phi), sin(psi)*sin(theta)*cos(phi)-cos(psi)*sin(phi), cos(theta)*cos(phi)] *...
            [0;0;u_Thrust_I];

== matlab function model_groundTethered/Plant/Tether_Kite_Tether_UAV_Dynamics_1P/UAV_Model/UAV_Dynamics ==
  data: x_dotdot_uav_trans output; omega_dot output; eta_dot output; Thrust input; m_uav parameter; g_vec parameter; x_UAV input; x_below_UAV input; x_dot_UAV input; x_dot_belowUAV input; c0 parameter; d0 parameter; l_s0 parameter; disturbance output; omega input; u_M input; J parameter; Jinv parameter; eta input
function [x_dotdot_uav_trans,omega_dot, eta_dot,  disturbance] = fcn(Thrust, m_uav, g_vec, x_UAV, x_below_UAV, x_dot_UAV, x_dot_belowUAV,...
    c0, d0, l_s0, omega, u_M, J,Jinv,eta )
%#codegen

%% Translational Dynamics
f_T_below = calcSpringDamperForce(c0, norm(x_UAV-x_below_UAV) , l_s0, d0, x_UAV-x_below_UAV, x_dot_UAV - x_dot_belowUAV, 1 );
disturbance = -f_T_below/m_uav;
%disturbance = 1/m_uav *[0;0;25] ;
x_dotdot_uav_trans = 1/m_uav * ( -1*f_T_below + Thrust - m_uav*g_vec + 0*[0;0;25]  ) ; % Drone dynamics

%% Rotational Dynamics 
p = omega(1); 
q = omega(2); 
r = omega(3); 
Ix = J(1,1); 
Iy = J(2,2); 
Iz = J(3,3); 

cross_coupling = [ Iy*q*r - Iz*q*r
                   Iz*p*r - Ix*p*r;
                   Ix*p*q - Iy*p*q];
% Bodyrate Dynamics
omega_dot = Jinv * ( cross_coupling + u_M ) ;  

% Attitude Dynamics
eta_dot = [1, sin(eta(1)) * tan(eta(2)), cos(eta(1)) * tan(eta(2)) ; 
0, cos(eta(1)), -sin(eta(1)); 
0, sin(eta(1))/cos(eta(2)), cos(eta(1))/cos(eta(2))] * omega ;

== matlab function model_groundTethered/Controller/Inner_Loop_Attitude/Reference_Model1/Reference Model 2nd order ==
  data: eta_c input; eta_r_dot output; A_r input; B_r input; eta_r_dotdot output; x input
function [eta_r_dot, eta_r_dotdot] = fcn(eta_c, A_r, B_r, x)


x_dot = A_r * x + B_r * eta_c;

eta_r_dot = x_dot(1:3);
eta_r_dotdot = x_dot(4:6);

== matlab function model_groundTethered/Flight_Path_Planner2/Reference_Dynamic_x1 ==
  data: x_cmd input; x_ref input; x_ref_dot output; t0 parameter; t1 parameter
function x_ref_dot = fcn(x_cmd, x_ref, t0, t1)

% a0 = 1;
% a1 = 5;

x_ref_dot = [0,1;
                -t0, -t1]*x_ref + [0;t0] * x_cmd;

== matlab function model_groundTethered/Flight_Path_Planner2/Reference_Dynamic_x2 ==
  data: x_cmd input; x_ref input; x_ref_dot output; t0 parameter; t1 parameter
function x_ref_dot = fcn(x_cmd, x_ref, t0, t1)

% a0 = 1;
% a1 = 5;

x_ref_dot = [0,1;
                -t0, -t1]*x_ref + [0;t0] * x_cmd;
